simulink model "RETINA_NEXUS_SYSTEM"  (R2026a)
settings: Solver=FixedStepDiscrete  StopTime=cfg.simulation_seconds  FixedStep=1
undefined symbols (not defined in the file): cfg, m, n
settings Model: Creator=kiran  LastModifiedBy=kiran

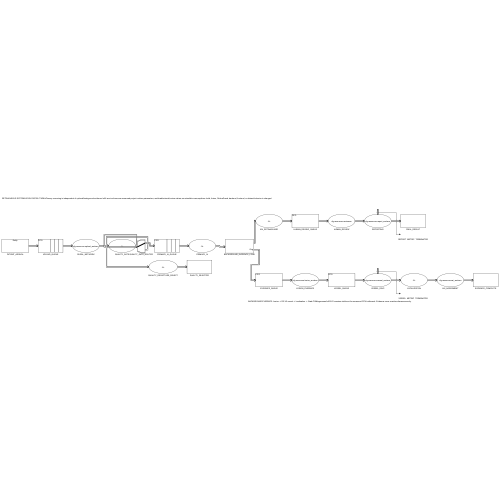
[thumbnail: Simulink's stored preview of the top-level diagram]
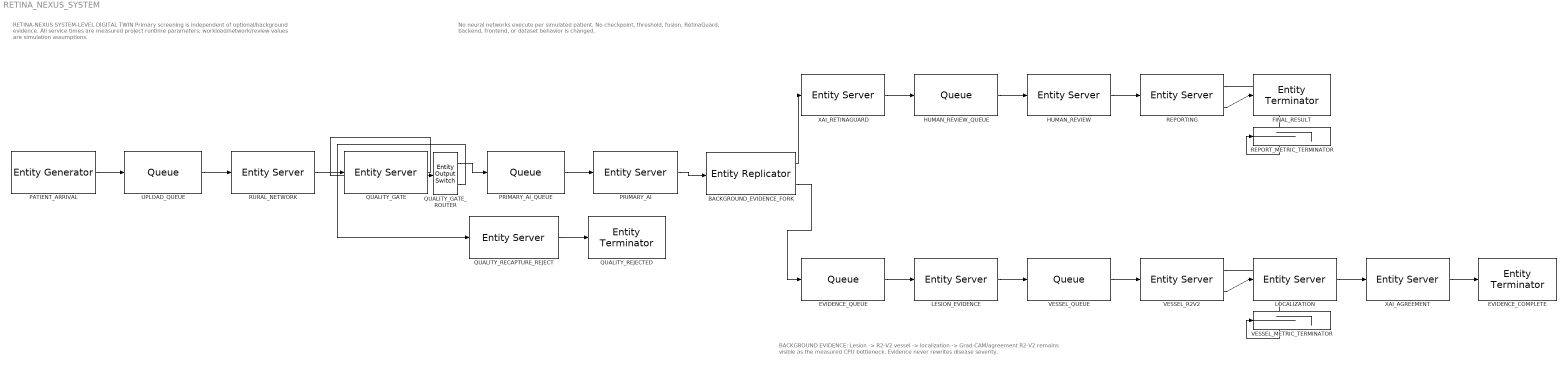
== system RETINA_NEXUS_SYSTEM ==
  note: RETINA-NEXUS SYSTEM-LEVEL DIGITAL TWIN\nPrimary screening is independent of optional/background evidence.\nAll service times are measured project runtime parameters; workload/network/review values are simulation assumptions.
  note: BACKGROUND EVIDENCE: Lesion -> R2-V2 vessel -> localization -> Grad-CAM/agreement\nR2-V2 remains visible as the measured CPU bottleneck. Evidence never rewrites disease severity.
  note: No neural networks execute per simulated patient.\nNo checkpoint, threshold, fusion, RetinaGuard, backend, frontend, or dataset behavior is changed.
  BACKGROUND_EVIDENCE_FORK : EntityReplicator  InputPortMessageModes=m  OutputPortMessageModes=m,m
  EVIDENCE_COMPLETE : EntityTerminator  InputPortMessageModes=m
  EVIDENCE_QUEUE : Queue  InputPortMessageModes=m  OutputPortMessageModes=m  Capacity=inf
  FINAL_RESULT : EntityTerminator  InputPortMessageModes=m
  HUMAN_REVIEW : EntityServer  InputPortMessageModes=m  OutputPortMessageModes=m  Capacity=cfg.resources.reviewers  ServiceTimeValue=cfg.review_time_minutes*60
  HUMAN_REVIEW_QUEUE : Queue  InputPortMessageModes=m  OutputPortMessageModes=m  Capacity=inf
  LESION_EVIDENCE : EntityServer  InputPortMessageModes=m  OutputPortMessageModes=m  Capacity=cfg.resources.lesion_workers  ServiceTimeValue=cfg.active_service_times.lesion
  LOCALIZATION : EntityServer  InputPortMessageModes=m  OutputPortMessageModes=m  Capacity=cfg.resources.localization_workers  ServiceTimeValue=cfg.active_service_times.localization
  PATIENT_ARRIVAL : EntityGenerator  OutputPortMessageModes=m  Period=cfg.interarrival_seconds  GenerateEntityAtSimulationStart=off  AttributeName=QualityPort  AttributeInitialValue=1+(rand(1,1)<cfg.quality_rejection_rate)  EntityType=Structured  EntityTypeName=Entity
  PRIMARY_AI : EntityServer  InputPortMessageModes=m  OutputPortMessageModes=m  Capacity=cfg.resources.classifier_workers  ServiceTimeValue=cfg.active_service_times.classification
  PRIMARY_AI_QUEUE : Queue  InputPortMessageModes=m  OutputPortMessageModes=m  Capacity=inf
  QUALITY_GATE : EntityServer  InputPortMessageModes=m  OutputPortMessageModes=m  Capacity=cfg.resources.acquisition_workers  ServiceTimeValue=cfg.active_service_times.quality_gate
  QUALITY_GATE_ROUTER : EntityOutputSwitch  InputPortMessageModes=m  OutputPortMessageModes=m,m  SwitchingCriterion=From attribute  SwitchAttributeName=QualityPort
  QUALITY_RECAPTURE_REJECT : EntityServer  InputPortMessageModes=m  OutputPortMessageModes=m  Capacity=cfg.resources.acquisition_workers  ServiceTimeValue=cfg.active_service_times.capture
  QUALITY_REJECTED : EntityTerminator  InputPortMessageModes=m
  REPORTING : EntityServer  InputPortMessageModes=m  OutputPortMessageModes=n,m  Capacity=cfg.resources.report_workers  ServiceTimeValue=cfg.active_service_times.pdf  NumberEntitiesDeparted=on
      settings: OutputPortMap=o0,o9
  REPORT_METRIC_TERMINATOR : Terminator
  RURAL_NETWORK : EntityServer  InputPortMessageModes=m  OutputPortMessageModes=m  Capacity=cfg.resources.upload_workers  ServiceTimeValue=cfg.transmission_time_s
  UPLOAD_QUEUE : Queue  InputPortMessageModes=m  OutputPortMessageModes=m  Capacity=inf
  VESSEL_METRIC_TERMINATOR : Terminator
  VESSEL_QUEUE : Queue  InputPortMessageModes=m  OutputPortMessageModes=m  Capacity=inf
  VESSEL_R2V2 : EntityServer  InputPortMessageModes=m  OutputPortMessageModes=n,m  Capacity=cfg.resources.vessel_workers  ServiceTimeValue=cfg.active_service_times.vessel  NumberEntitiesDeparted=on
      settings: OutputPortMap=o0,o9
  XAI_AGREEMENT : EntityServer  InputPortMessageModes=m  OutputPortMessageModes=m  Capacity=cfg.resources.xai_workers  ServiceTimeValue=cfg.active_service_times.xai_agreement
  XAI_RETINAGUARD : EntityServer  InputPortMessageModes=m  OutputPortMessageModes=m  Capacity=cfg.resources.classifier_workers  ServiceTimeValue=cfg.active_service_times.retina_guard
  wires:
  PATIENT_ARRIVAL/1 -> UPLOAD_QUEUE/1
  UPLOAD_QUEUE/1 -> RURAL_NETWORK/1
  RURAL_NETWORK/1 -> QUALITY_GATE/1
  QUALITY_GATE/1 -> QUALITY_GATE_ROUTER/1
  QUALITY_GATE_ROUTER/1 -> PRIMARY_AI_QUEUE/1
  QUALITY_GATE_ROUTER/2 -> QUALITY_RECAPTURE_REJECT/1
  QUALITY_RECAPTURE_REJECT/1 -> QUALITY_REJECTED/1
  PRIMARY_AI_QUEUE/1 -> PRIMARY_AI/1
  PRIMARY_AI/1 -> BACKGROUND_EVIDENCE_FORK/1
  BACKGROUND_EVIDENCE_FORK/1 -> XAI_RETINAGUARD/1
  XAI_RETINAGUARD/1 -> HUMAN_REVIEW_QUEUE/1
  HUMAN_REVIEW_QUEUE/1 -> HUMAN_REVIEW/1
  HUMAN_REVIEW/1 -> REPORTING/1
  REPORTING/2 -> FINAL_RESULT/1
  BACKGROUND_EVIDENCE_FORK/2 -> EVIDENCE_QUEUE/1
  EVIDENCE_QUEUE/1 -> LESION_EVIDENCE/1
  LESION_EVIDENCE/1 -> VESSEL_QUEUE/1
  VESSEL_QUEUE/1 -> VESSEL_R2V2/1
  VESSEL_R2V2/2 -> LOCALIZATION/1
  LOCALIZATION/1 -> XAI_AGREEMENT/1
  XAI_AGREEMENT/1 -> EVIDENCE_COMPLETE/1
  REPORTING/1 -> REPORT_METRIC_TERMINATOR/1
  VESSEL_R2V2/1 -> VESSEL_METRIC_TERMINATOR/1
